simulink model "lab12_PE_Analysis"  (R2025a)
settings: Solver=VariableStepAuto  StartTime=0.0  StopTime=10.0  RelTol=1e-3
settings Model: Creator=hp  LastModifiedBy=hp

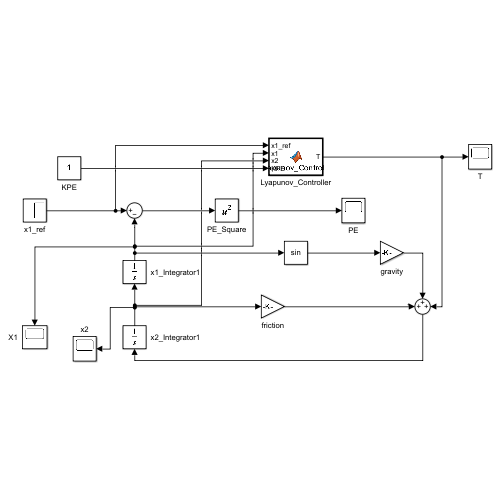
[thumbnail: Simulink's stored preview of the top-level diagram]
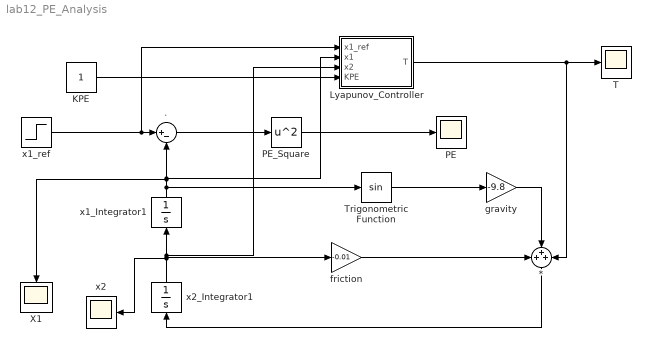
== system lab12_PE_Analysis ==
  * : Sum  Inputs=+++
  . : Sum  Inputs=|+-
  KPE : Constant
  Lyapunov_Controller : MATLAB Function  TreatAsAtomicUnit=on
  PE : Scope
      settings: ActiveDisplayYMinimum=-0.124999999999999  ActiveDisplayYMaximum=1.125  DataLoggingVariableName=ScopeData3
  PE_Square : Math  Operator=square
  T : Scope
      settings: ActiveDisplayYMinimum=-1  ActiveDisplayYMaximum=1  DataLoggingVariableName=ScopeData2
  Trigonometric Function : Trigonometry
  X1 : Scope
      settings: ActiveDisplayYMinimum=-0.150917494972421  ActiveDisplayYMaximum=1.3582574547517892
  friction : Gain  Gain=-0.01
  gravity : Gain  Gain=-9.8
  x1_Integrator1 : Integrator
  x1_ref : Step  Time=0  SampleTime=0
  x2 : Scope
      settings: ActiveDisplayYMinimum=-0.57771221459797317  ActiveDisplayYMaximum=2.0310054536122935
  x2_Integrator1 : Integrator
  wires:
  x1_ref/1 -> Lyapunov_Controller/1(x1_ref), ./1
  ./1 -> PE_Square/1
  x2_Integrator1/1 -> Lyapunov_Controller/3(x2), x1_Integrator1/1, friction/1, x2/1
  x1_Integrator1/1 -> Lyapunov_Controller/2(x1), ./2, X1/1, Trigonometric Function/1
  Trigonometric Function/1 -> gravity/1
  */1 -> x2_Integrator1/1
  friction/1 -> */1
  gravity/1 -> */2
  Lyapunov_Controller/1(T) -> T/1, */3
  PE_Square/1 -> PE/1
  KPE/1 -> Lyapunov_Controller/4(KPE)

== matlab function lab12_PE_Analysis/Lyapunov_Controller ==
  data: x1_ref input; T output; x1 input; x2 input; KPE input
function T = Lyapunov_Controller(x1_ref, x1, x2, KPE)

Kd = 2;

e = x1_ref - x1;

T = 9.8*sin(x1) + 0.01*x2 ...
    + KPE*e ...
    - Kd*x2;

end
